simulink subsystem "States"  (R2024b)
settings: Solver=VariableStepAuto  StartTime=0.0  StopTime=10.0  RelTol=1e-3
settings Model: Creator=JesseJabezArendse  LastModifiedBy=JesseJabezArendse

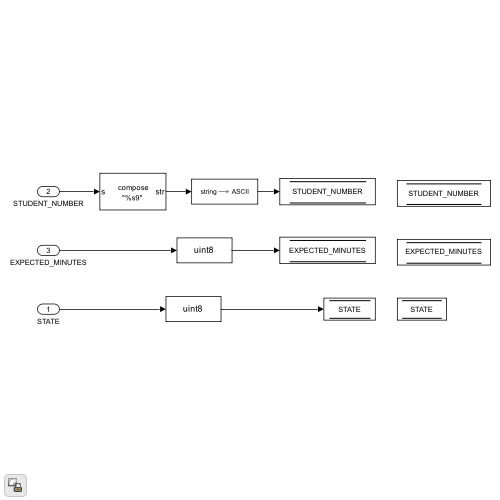
[thumbnail: Simulink's stored preview of the top-level diagram]
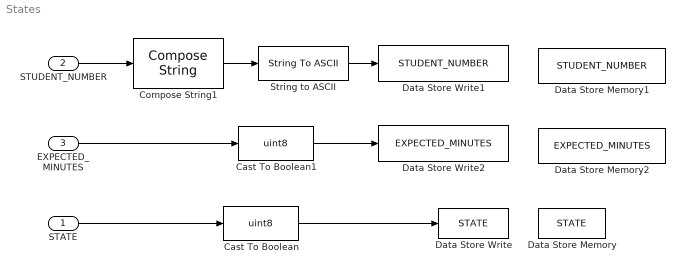
== system States ==
  STATE : Inport
  STUDENT_NUMBER : Inport  Port=2
  EXPECTED_MINUTES : Inport  Port=3
  Cast To Boolean : DataTypeConversion  OutDataTypeStr=uint8  SaturateOnIntegerOverflow=off  RndMeth=Floor
  Cast To Boolean1 : DataTypeConversion  OutDataTypeStr=uint8  SaturateOnIntegerOverflow=off  RndMeth=Floor
  Compose String1 : ComposeString  Format="\"%s9\""
  Data Store Memory : DataStoreMemory  DataStoreName=STATE  WriteAfterWriteMsg=warning  ShowAdditionalParam=off  OutDataTypeStr=uint8  Dimensions=1
  Data Store Memory1 : DataStoreMemory  DataStoreName=STUDENT_NUMBER  WriteAfterWriteMsg=warning  ShowAdditionalParam=off  Dimensions=9
  Data Store Memory2 : DataStoreMemory  DataStoreName=EXPECTED_MINUTES  WriteAfterWriteMsg=warning  ShowAdditionalParam=off  OutDataTypeStr=uint8  Dimensions=1
  Data Store Write : DataStoreWrite  DataStoreName=STATE  IndexOptions=Index vector (dialog)  Indices=1  OutputSizes=1
  Data Store Write1 : DataStoreWrite  DataStoreName=STUDENT_NUMBER  IndexOptions=Index vector (dialog)  Indices=1  OutputSizes=1
  Data Store Write2 : DataStoreWrite  DataStoreName=EXPECTED_MINUTES  IndexOptions=Index vector (dialog)  Indices=1  OutputSizes=1
  String to ASCII : StringToASCII  OutputVectorSize=9
  wires:
  STATE/1 -> Cast To Boolean/1
  Cast To Boolean/1 -> Data Store Write/1
  STUDENT_NUMBER/1 -> Compose String1/1
  EXPECTED_MINUTES/1 -> Cast To Boolean1/1
  Cast To Boolean1/1 -> Data Store Write2/1
  Compose String1/1 -> String to ASCII/1
  String to ASCII/1 -> Data Store Write1/1
